simulink model "bicycle_center_of_gravity_simulation"  (R2018a)
settings: Solver=FixedStepAuto  StartTime=0.0  StopTime=40  FixedStep=1e-2  RelTol=1e-3
undefined symbols (not defined in the file or in its folder): Model
settings Model: Creator=ASUS PRO  LastModifiedBy=ASUS PRO

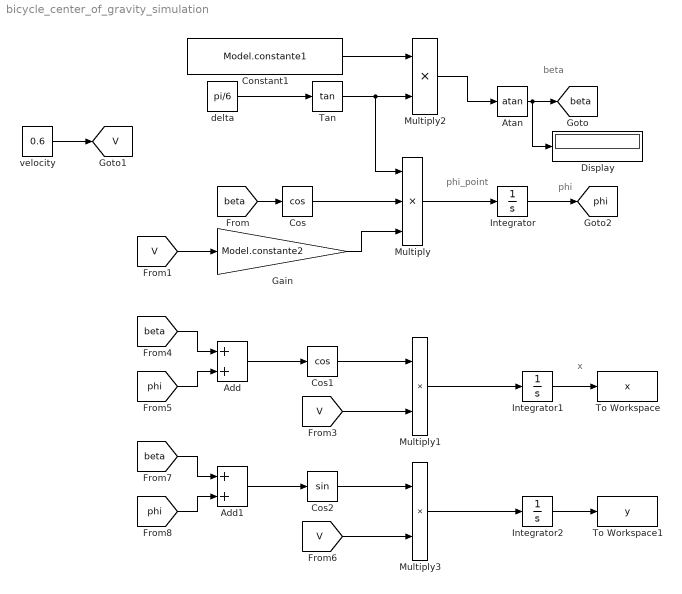
== system bicycle_center_of_gravity_simulation ==
  note: x
  note: beta
  note: phi_point
  note: phi
  Add : Sum
  Add1 : Sum
  Atan : Trigonometry  Operator=atan
  Constant1 : Constant  Value=Model.constante1
  Cos : Trigonometry  Operator=cos
  Cos1 : Trigonometry  Operator=cos
  Cos2 : Trigonometry
  Display : Display
  Gain : Gain  Gain=Model.constante2
  Integrator : Integrator
  Integrator1 : Integrator
  Integrator2 : Integrator
  Multiply : Product  Inputs=3
  Multiply1 : Product
  Multiply2 : Product
  Multiply3 : Product
  Tan : Trigonometry  Operator=tan
  To Workspace : ToWorkspace  VariableName=x  SampleTime=-1
  To Workspace1 : ToWorkspace  VariableName=y  SampleTime=-1
  delta : Constant  Value=pi/6
  "velocity " : Constant  Value=0.6
  tag scope: V=global, beta=global, phi=global
  wires:
  Integrator/1 -> [phi]
  Multiply/1 -> Integrator/1
  Cos/1 -> Multiply/2
  Multiply2/1 -> Atan/1
  delta/1 -> Tan/1
  Tan/1 -> Multiply/1, Multiply2/2
  Constant1/1 -> Multiply2/1
  [beta] -> Cos/1
  Gain/1 -> Multiply/3
  "velocity "/1 -> [V]
  [V] -> Gain/1
  Integrator1/1 -> To Workspace/1
  Multiply1/1 -> Integrator1/1
  Cos1/1 -> Multiply1/1
  [V] -> Multiply1/2
  Add/1 -> Cos1/1
  [beta] -> Add/1
  [phi] -> Add/2
  [phi] -> Add1/2
  [beta] -> Add1/1
  Add1/1 -> Cos2/1
  [V] -> Multiply3/2
  Cos2/1 -> Multiply3/1
  Multiply3/1 -> Integrator2/1
  Integrator2/1 -> To Workspace1/1
  Atan/1 -> [beta], Display/1
